simulink model "problem_finl"  (R2020b)
settings: Solver=VariableStepAuto  StartTime=0.0  StopTime=10.0  RelTol=1e-3
settings Model: Creator=Admin  LastModifiedBy=HP

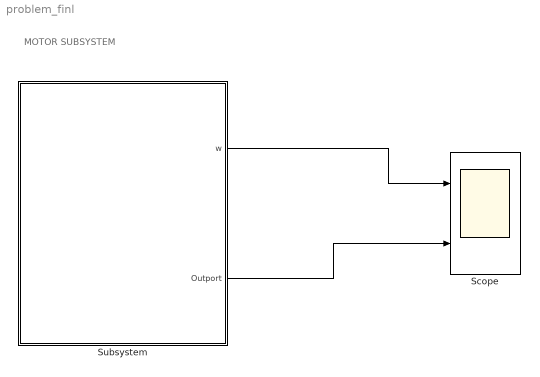
== system problem_finl ==
  note: MOTOR SUBSYSTEM
  Scope : Scope  NumInputPorts=2
  Subsystem : Subsystem
  wires:
  Subsystem/1(w) -> Scope/1
  Subsystem/2(Outport) -> Scope/2

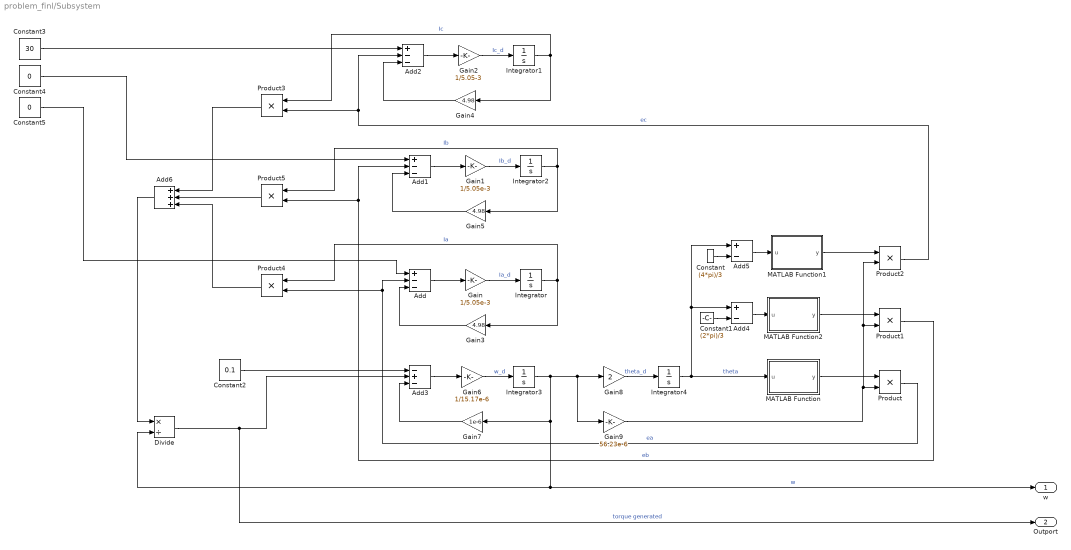
== system problem_finl/Subsystem ==
  Add : Sum  Inputs=+--
  Add1 : Sum  Inputs=+--
  Add2 : Sum  Inputs=+--
  Add3 : Sum  Inputs=-+-
  Add4 : Sum  Inputs=+-
  Add5 : Sum  Inputs=+-
  Add6 : Sum  Inputs=+++
  Constant : Constant  Value=(4*pi)/3
  Constant1 : Constant  Value=(2*pi)/3
  Constant2 : Constant  Value=0.1
  Constant3 : Constant  Value=30
  Constant4 : Constant  Value=0
  Constant5 : Constant  Value=0
  Divide : Product  Inputs=*/
  Gain : Gain  Gain=1/5.05e-3
  Gain1 : Gain  Gain=1/5.05e-3
  Gain2 : Gain  Gain=1/5.05-3
  Gain3 : Gain  Gain=4.98
  Gain4 : Gain  Gain=4.98
  Gain5 : Gain  Gain=4.98
  Gain6 : Gain  Gain=1/15.17e-6
  Gain7 : Gain  Gain=1e-6
  Gain8 : Gain  Gain=2
  Gain9 : Gain  Gain=56.23e-6
  Integrator{,1..2,4} (4 alike) : Integrator
  Integrator3 : Integrator  InitialCondition=1
  MATLAB Function : MATLAB Function  TreatAsAtomicUnit=on
  MATLAB Function1 : MATLAB Function  TreatAsAtomicUnit=on
  MATLAB Function2 : MATLAB Function  TreatAsAtomicUnit=on
  Product{,1..5} (6 alike) : Product
  w : Outport
  Outport : Outport  Port=2
  wires:
  Product3/1 -> Add6/1
  Add3/1 -> Gain6/1
  Add/1 -> Gain/1
  Constant3/1 -> Add2/1
  Gain2/1 -> Integrator1/1  "Ic_d"
  Integrator/1 -> Gain3/1, Product4/1  "Ia"
  Constant1/1 -> Add4/2
  Gain9/1 -> Product2/2, Product1/2, Product/2
  Add4/1 -> MATLAB Function2/1(u)
  Add5/1 -> MATLAB Function1/1(u)
  Integrator4/1 -> MATLAB Function/1(u), Add5/1, Add4/1  "theta"
  Constant5/1 -> Add/1
  Constant2/1 -> Add3/1
  Integrator2/1 -> Gain5/1, Product5/1  "Ib"
  Product/1 -> Product4/2, Add/2  "ea"
  Product2/1 -> Add2/2, Product3/2  "ec"
  Divide/1 -> Outport/1, Add3/2  "torque generated"
  Add1/1 -> Gain1/1
  Constant4/1 -> Add1/1
  MATLAB Function2/1(y) -> Product1/1
  MATLAB Function/1(y) -> Product/1
  Gain/1 -> Integrator/1  "Ia_d"
  Gain1/1 -> Integrator2/1  "Ib_d"
  MATLAB Function1/1(y) -> Product2/1
  Gain8/1 -> Integrator4/1  "theta_d"
  Product4/1 -> Add6/3
  Gain6/1 -> Integrator3/1  "w_d"
  Gain7/1 -> Add3/3
  Gain3/1 -> Add/3
  Integrator1/1 -> Gain4/1, Product3/1  "Ic"
  Integrator3/1 -> Gain8/1, Gain9/1, Gain7/1, w/1, Divide/2  "w"
  Gain5/1 -> Add1/3
  Constant/1 -> Add5/2
  Product1/1 -> Product5/2, Add1/2  "eb"
  Add2/1 -> Gain2/1
  Add6/1 -> Divide/1
  Product5/1 -> Add6/2
  Gain4/1 -> Add2/3

== matlab function problem_finl/Subsystem/MATLAB Function ==
  data: u input; y output
function y = fcn(u)

if (u>=0 && u<((2*pi)/3))
    y = 1;
elseif(u>=((2*pi)/3) && u<pi)
    y = 1-(6/pi*(u-((2*pi)/3)));
elseif(u>=pi && u<((5*pi)/3))
    y = -1;
else
    y = -1+(6/pi*(u-((5*pi)/3)));
end
end

== matlab function problem_finl/Subsystem/MATLAB Function2 ==
  data: u input; y output
function y = fcn(u)

if (u>=0 && u<((2*pi)/3))
    y = 1;
elseif(u>=((2*pi)/3) && u<pi)
    y = 1-(6/pi*(u-((2*pi)/3)));
elseif(u>=pi && u<((5*pi)/3))
    y = -1;
else
    y = -1+(6/pi*(u-((5*pi)/3)));
end
end

== matlab function problem_finl/Subsystem/MATLAB Function1 ==
  data: u input; y output
function y = fcn(u)

if (u>=0 && u<((2*pi)/3))
    y = 1;
elseif(u>=((2*pi)/3) && u<pi)
    y = 1-(6/pi*(u-((2*pi)/3)));
elseif(u>=pi && u<((5*pi)/3))
    y = -1;
else
    y = -1+(6/pi*(u-((5*pi)/3)));
end
end
